simulink model "Problem8"  (R2020a)
settings: Solver=FixedStepAuto  StartTime=0.0  StopTime=10.0  RelTol=1e-3
settings Model: Creator=tnradm  LastModifiedBy=tnradm

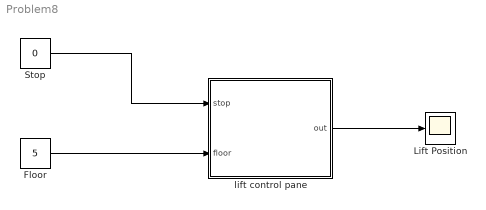
== system Problem8 ==
  Floor : Constant  Value=5
  Lift Position : Scope
  Stop : Constant  Value=0
  lift control pane : Stateflow chart  TreatAsAtomicUnit=on
  wires:
  Floor/1 -> lift control pane/2(floor)
  Stop/1 -> lift control pane/1(stop)
  lift control pane/1(out) -> Lift Position/1

== stateflow chart Problem8/lift control pane ==
  state Start
  state Normal_op
    (default) -> (junction 12) : [floor>0&&stop==0]
    (junction 12) -> (junction 24) [order 1] : [floor==1]{out=floor}
    (junction 12) -> (junction 28) [order 2] : [floor==2]{out=floor}
    (junction 12) -> (junction 34) [order 5] : [floor==5]{out=floor}
    (junction 12) -> (junction 30) [order 3] : [floor==3]{out=floor}
    (junction 12) -> (junction 32) [order 4] : [floor==4]{out=floor}
  state Stop
    entry:stp();
    exit:
  (default) -> Start
  Start -> Stop [order 2] : [stop==1]
  Start -> Normal_op [order 1] : [stop==0]
  data: stop input; floor input; out output
  function stp:
    | function stp
    |     out=floor;
